simulink model "PKM_Planar_Testbench_2018"  (R2024a)
settings: Solver=FixedStepDiscrete  StartTime=0.0  StopTime=inf  FixedStep=param.t_sample  RelTol=1e-3
undefined symbols (not defined in the file or in its folder): max_qa, min_qa, param, slave3
libraries: Cust_Library_planarPKM x54, simulink_extras x27, dspswit3 x24, simulink x22, etherlab_lib x12
(part 3 of 6)

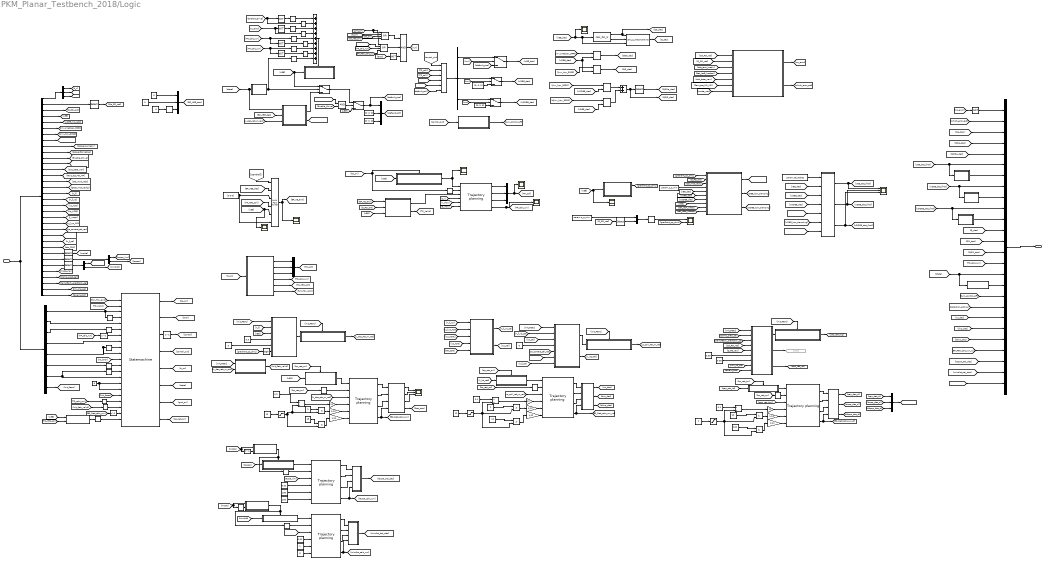
== system PKM_Planar_Testbench_2018/Logic ==
  note: Processing of logical signals
  note: xE: Desired platform pose
  note: Trajectory planning for activated inequality constraints
  note: Inverse kinematics
  note: Safety functions
  note: Platform Coordinate selection
  note: Structure opening for clamping contacts
  note: Retraction via contact coordinates
  note: Trajectory
  note: Check whether the EE target pose is in the operational space
      | and the corresponding joint angles are in the joint space
  note: Selection of the target EE pose for trajectoy planning
  note: For the PTP/CTP movement: An acceleration trapezoidal profile is calculated using the EE end target pose and the EE actual pose,
      | to determine the target EE pose, target EE velocity and target EE acceleration (all three in BP_target)
  note: Clamping reaction by platform reorientation
  note: Retraction movement via platform coordinates
  Data : Inport
  AND : Logic  AllPortsSameDT=off  OutDataTypeStr=boolean
  AND1 : Logic  Operator=OR  Inputs=4  AllPortsSameDT=off  OutDataTypeStr=boolean
  AND2 : Logic  Inputs=3  AllPortsSameDT=off  OutDataTypeStr=boolean
  AND3 : Logic  Operator=OR  Inputs=4  AllPortsSameDT=off  OutDataTypeStr=boolean
  Add : Sum  Inputs=9
  Add3 : Sum
  Angle clamping : Constant  Value=param.q_p_min  SampleTime=-1
  Angle clamping1 : Constant  Value=param.q_p_min  SampleTime=-1
  Bus Creator : BusCreator  Inputs=26
  Bus Selector : BusSelector  OutputSignals=Controlpanel.tv_vmax_amax,Kinematics_currentValues.Qa_rad_m,Kinematics_currentValues.Q_rad,Kinematics_currentValues.xEE_m_rad,Differential kinematics - current values.xDEE_ms_rads,Differential kinematics - current values.Jinv_hredqax,Differential kinematics - current values.Jinv_hqx,Differential kinematics - current values.dJinv_hqx,Differential kinematics - current values.det_JacA_hredx,Differential kinematics - current values.det_JacB_hredqa,Controlpanel.Enable_Drive,Controlpanel.Enable_PDControl,Beobachter.obs_beta_nan,Beobachter.rx,Differential kinematics - current values.QD_mod_rads,Differential kinematics - current values.QDD_mod_radss,Beobachter.Wirklinie_Fext_mP,Beobachter.Wirklinie_Fext_xp,Beobachter.xp_KS0,Beobachter.xp_KSGj,Beobachter.J_xpqa,Beobachter.n_f_xp_KS0,Beobachter.qa_contact_sel_rad,Beobachter.predbody_sel,Beobachter.n_f_qa,Controlpanel.retr_CS0,PD_Controller.mode_h_rrlevel_rrrueck,PD_Controller.kappa_lim_soll_ist,PD_Controller.min_dist_lim_soll_ist,PD_Controller.mode_nan,Beobachter.clamping_predicted,Beobachter.clampingChain_predicted,Differential kinematics - current values.Jinv_hqx_dq_dqa,Beobachter.tauext_obs
  Bus Selector1 : BusSelector  OutputSignals=Controlpanel.Drive_to_Position,Controlpanel.EMERGENCY_OFF,Controlpanel.GUI_started,State Variables.Controlword,Controlpanel.Drive_to_Homepose,Controlpanel.Enable_Drive,Controlpanel.Drive_trajectory,Beobachter.Init_Reaktion
  Clamping reaction : MATLAB Function  TreatAsAtomicUnit=on
  Constant : Constant  Value=[0;0;0]  SampleTime=-1
  Constant1 : Constant  Value=param.sel_redres  SampleTime=-1
  Constant10 : Constant  Value=150  SampleTime=-1
  Constant12 : Constant  Value=0  SampleTime=-1
  Constant14 : Constant  Value=150  SampleTime=-1
  Constant16 : Constant  SampleTime=-1
  Constant17 : Constant  Value=5  SampleTime=-1
  Constant18 : Constant  Value=0.01  SampleTime=-1
  Constant{4..5,7..8} (4 alike) : Constant  Value=[0; 0; 0]  SampleTime=-1
  Constant9 : Constant  Value=0.01  SampleTime=-1
  Degrees to Radians1 : simulink_extras/Transformations/Degrees to Radians
  Delay{,1..3,7,9,14..15} (8 alike) : Delay  DelayLength=1
  Demux1 : Demux  Outputs=2
  Demux2 : Demux  Outputs=2
  Demux3 : Demux  Outputs=3
  Demux4 : Demux  Outputs=3
  Divide : Product  Inputs=*/
  Divide1 : Product  Inputs=*/
  Divide2 : Product  Inputs=*/
  Edge Detector{1..6,8..21} (20 alike) : dspswit3/Edge Detector  InputProcessing=Columns as channels (frame based)
  Gain10 : Gain  Gain=12
  Gain{11..12,14..15,21..22} (6 alike) : Gain  Gain=1/12
  Gain13 : Gain  Gain=12
  Gain20 : Gain  Gain=12
  Goto106 : Goto  Commented=on  GotoTag=Jqap
  Gradient calculation : MATLAB Function  TreatAsAtomicUnit=on
  Hold Configuration after enabling1 : Subsystem  TreatAsAtomicUnit=on
  Hold Configuration after enabling2 : Subsystem  TreatAsAtomicUnit=on
  Hold Configuration after enabling3 : Subsystem  TreatAsAtomicUnit=on
  Hold Configuration after enabling4 : Subsystem  TreatAsAtomicUnit=on
  Hold Configuration after enabling5 : Subsystem  TreatAsAtomicUnit=on
  Hold Configuration after enabling6 : Subsystem  TreatAsAtomicUnit=on
  Hold Configuration after enabling7 : Subsystem  TreatAsAtomicUnit=on
  Hold Configuration after enabling8 : Subsystem  TreatAsAtomicUnit=on
  Hold Configuration after enabling9 : Subsystem  TreatAsAtomicUnit=on
  "Hold initial position as target value for PD_Controller " : Subsystem  TreatAsAtomicUnit=on
  MATLAB Function : MATLAB Function  TreatAsAtomicUnit=on
  MATLAB Function1 : MATLAB Function  TreatAsAtomicUnit=on
  MATLAB Function11 : MATLAB Function  TreatAsAtomicUnit=on
  MATLAB Function12 : MATLAB Function  TreatAsAtomicUnit=on
  MATLAB Function13 : MATLAB Function  TreatAsAtomicUnit=on
  MATLAB Function14 : MATLAB Function  TreatAsAtomicUnit=on
  MATLAB Function15 : MATLAB Function  TreatAsAtomicUnit=on
  MATLAB Function16 : MATLAB Function  TreatAsAtomicUnit=on
  MATLAB Function17 : MATLAB Function  TreatAsAtomicUnit=on
  MATLAB Function18 : MATLAB Function  TreatAsAtomicUnit=on
  MATLAB Function19 : MATLAB Function  TreatAsAtomicUnit=on
  MATLAB Function2 : MATLAB Function  TreatAsAtomicUnit=on
  MATLAB Function20 : MATLAB Function  TreatAsAtomicUnit=on
  MATLAB Function21 : MATLAB Function  TreatAsAtomicUnit=on
  MATLAB Function22 : MATLAB Function  TreatAsAtomicUnit=on
  MATLAB Function23 : MATLAB Function  TreatAsAtomicUnit=on
  MATLAB Function3 : MATLAB Function  TreatAsAtomicUnit=on
  MATLAB Function4 : MATLAB Function  TreatAsAtomicUnit=on
  MATLAB Function7 : MATLAB Function  TreatAsAtomicUnit=on
  MATLAB Function8 : MATLAB Function  TreatAsAtomicUnit=on
  MatrixMultiply{8..11} (4 alike) : Product  Multiplication=Matrix(*)
  Multiport Switch : MultiPortSwitch  Inputs=4  DataPortForDefault=Additional data port  DiagnosticForDefault=None  SaturateOnIntegerOverflow=off  InputSameDT=off
  Multiport Switch1 : MultiPortSwitch  Inputs=4  DataPortForDefault=Additional data port  DiagnosticForDefault=None  SaturateOnIntegerOverflow=off  InputSameDT=off
  Mux{,1,3..4,9} (5 alike) : Mux  Inputs=3
  Mux2 : Mux  Inputs=2
  NOT{,1..5} (6 alike) : Logic  Operator=NOT  AllPortsSameDT=off  OutDataTypeStr=boolean
  PHIE : Constant  Value=0  SampleTime=-1
  Radians to Degrees : simulink_extras/Transformations/Radians to Degrees
  Safety functions : Subsystem
  Saturation : Saturate  UpperLimit=12  LowerLimit=1
  Saturation1 : Saturate  UpperLimit=12  LowerLimit=1
  Saturation2 : Saturate  UpperLimit=12  LowerLimit=1
  Scope{,1,4,12,14,23,31} (7 alike) : Scope
  Scope27 : Scope  NumInputPorts=2
  Scope28 : Scope  NumInputPorts=3
  Scope48 : Scope  NumInputPorts=3
  Selector : Selector  InputPortWidth=9  IndexOptions=Index vector (dialog)  Indices=[2 5 8]  OutputSizes=1
  Selector2 : Selector  InputPortWidth=9  IndexOptions=Index vector (dialog)  Indices=[1 4 7]  OutputSizes=1
  Selector3 : Selector  InputPortWidth=4  IndexOptions=Index vector (dialog)  Indices=[1 2 3]  OutputSizes=1
  Selector5 : Selector  InputPortWidth=5  IndexOptions=Index vector (dialog)  Indices=[1]  OutputSizes=1
  Selector6 : Selector  InputPortWidth=4  IndexOptions=Index vector (dialog)  Indices=[1 4]  OutputSizes=1
  Selector7 : Selector  InputPortWidth=4  IndexOptions=Index vector (dialog)  Indices=[1 4]  OutputSizes=1
  Sign1 : Signum
  Statemachine : Cust_Library_planarPKM/Statemachine  SystemSampleTime=-1  VariantActivationTime=update diagram  AllowFlexibleInterface=on  Latency=0  AutoFrameSizeCalculation=off
  Switch{2..6} (5 alike) : Switch  Criteria=u2 > Threshold  SaturateOnIntegerOverflow=off  InputSameDT=off
  Trajectory : Subsystem
  Trajectory planning{,1..5} (6 alike) : Cust_Library_planarPKM/Trajectory planning
  Validation of the EE end target pose : Subsystem
  XE : Constant  Value=0  SampleTime=-1
  YE : Constant  Value=0  SampleTime=-1
  amax : Constant  Value=15  SampleTime=-1
  amax1 : Constant  Value=10  SampleTime=-1
  amax2 : Constant  Value=100  SampleTime=-1
  bp_rueck : Constant  Value=12  SampleTime=-1
  bp_rueck2 : Constant  Value=12  SampleTime=-1
  calc_full_ik : Cust_Library_planarPKM/calc_full_ik  psi_j=param.psi_j  beta_j=param.beta_j  r_fixPlat_j=param.r_fixPlat_j  r_mobPlat_j=param.r_mobPlat_j  l_all_id=param.l_all_id
  calc_q_rotConstraints : Cust_Library_planarPKM/calc_q_rotConstraints  psi_j=param.psi_j
  d_retr_cl1 : Constant  Value=0.05  SampleTime=-1
  d_retr_cl2 : Constant  Value=0.05  SampleTime=-1
  d_retr_m : Constant  Value=0.3  SampleTime=-1
  d_retr_m1 : Constant  Value=0  SampleTime=-1
  isStandstill : MATLAB Function  TreatAsAtomicUnit=on
  mult{,1..5} (6 alike) : Product  Inputs=**
  phi_retr_deg : Constant  Value=0  SampleTime=-1
  tp_retr1 : Constant  SampleTime=-1
  tv : Constant  Value=0.2  SampleTime=-1
  tv1 : Constant  Value=0.1  SampleTime=-1
  tv2 : Constant  Value=0.1  SampleTime=-1
  vmax : Constant  Value=2  SampleTime=-1
  vmax1 : Constant  Value=2  SampleTime=-1
  vmax2 : Constant  Value=20  SampleTime=-1
  Out1 : Outport
  wires:
  Data/1 -> Bus Selector/1, Bus Selector1/1
  [TP_Valid] -> Statemachine/2
  Bus Selector1/1 -> Statemachine/3, Edge Detector5/1  "<Drive_to_Position>"
  Bus Selector1/2 -> Statemachine/5  "<EMERGENCY_OFF>"
  [TP_calc_run] -> Delay/1
  Bus Selector1/4 -> Statemachine/8  "<Controlword>"
  Bus Selector1/5 -> Statemachine/10, Edge Detector6/1  "<Drive_to_Homepose>"
  Bus Creator/1 -> Out1/1  "Logical data"
  Delay/1 -> Statemachine/7  "bp_calc_run"
  [no_error] -> Statemachine/11  "err"
  [Qa_des] -> Bus Creator/3  "Qa_des_rad"
  [QDa_des] -> Bus Creator/4  "QDa_des_rads"
  [QDDa_des] -> Bus Creator/5  "QDDa_des_radss"
  [xEE_des_final] -> MATLAB Function/1(u), Bus Creator/6  "xEE_des_m_rad"
  [xDEE_des_final] -> MATLAB Function2/1(u), Bus Creator/8  "xDEE_des_ms_rads"
  [xDDEE_des_final] -> MATLAB Function3/1(u), Bus Creator/10  "xDDEE_des_mss_radss"
  [TP_calc_run] -> Bus Creator/15  "TP_isCalculating"
  [Q_des] -> Bus Creator/12  "Q_des_rad"
  [QD_des] -> Bus Creator/13  "QD_des_rads"
  [QDD_des] -> Bus Creator/14  "QDD_des_radss"
  Statemachine/1 -> [bp_on]  "bp_on"
  Statemachine/2 -> [error]  "error"
  Bus Selector/1 -> Demux3/1  "<tv_vmax_amax>"
  Demux3/1 -> [t_v]  "t_v"
  Demux3/2 -> [v_max]  "v_max"
  Demux3/3 -> [a_max]  "a_max"
  Bus Selector1/7 -> Statemachine/14, Edge Detector1/1  "<Drive_trajectory>"
  [TR_calc_run] -> Delay1/1
  Statemachine/5 -> [tr_on]  "tr_on"
  Delay1/1 -> Statemachine/18
  [xEE] -> MATLAB Function1/1(EE_act)
  [TR_XE0_soll] -> MATLAB Function1/2(vec_traj_0)
  [full_TR_valid] -> Statemachine/1
  Statemachine/4 -> [control_out]  "control_out"
  Statemachine/3 -> Delay3/1
  MATLAB Function1/1(TR_in_starting_pos) -> Delay2/1
  Delay2/1 -> Statemachine/21  "tr_in_starting_pos"
  Delay3/1 -> [control]  "control"
  Statemachine/6 -> [state]  "state"
  [state] -> isStandstill/1(u), Bus Creator/16  "state"
  Bus Selector/2 -> Selector3/1  "<Qa_rad_m>"
  Bus Selector1/3 -> Edge Detector4/1  "<GUI_started>"
  Edge Detector4/1 -> Statemachine/6  "GUI_started"
  Edge Detector5/1 -> Statemachine/4  "target_run_trig"
  Edge Detector6/1 -> Statemachine/9  "home_run_trig"
  Edge Detector1/1 -> Statemachine/13
  Bus Selector1/6 -> Edge Detector3/1  "<Enable_Drive>"
  Edge Detector3/1 -> Statemachine/12  "enable_drive"
  Mux4/1 -> [BP_XEE_des]
  PHIE/1 -> Degrees to Radians1/1
  Degrees to Radians1/1 -> Mux4/3
  YE/1 -> Mux4/2
  XE/1 -> Mux4/1
  Bus Selector/4 -> [xEE]  "<xEE_m_rad>"
  [control] -> Multiport Switch/1
  [BP_XEE_des] -> Multiport Switch/2
  Multiport Switch/1 -> [BP_XE_end], Scope12/1
  [TR_XE0_soll] -> Multiport Switch/4
  [xEE] -> Scope14/1, Multiport Switch/5
  Mux/1 -> Scope/1, [TP_soll]  "soll_BP"
  Validation of the EE end target pose/2(BP_valid) -> [TP_Valid]
  Trajectory planning/1 -> Mux/1
  [a_max] -> Trajectory planning/6
  Edge Detector2/1 -> Trajectory planning/2  "enable_bp"
  Hold Configuration after enabling1/1("vec_x_0_Startposition ") -> Trajectory planning/1, Scope4/1
  [t_v] -> Trajectory planning/4
  [bp_on] -> Hold Configuration after enabling1/Trigger, Edge Detector2/1  "enable_bp"
  [v_max] -> Trajectory planning/5
  [xEE] -> Hold Configuration after enabling1/1(Theta_ist)
  Validation of the EE end target pose/1(XE_end) -> Trajectory planning/3
  Trajectory planning/4 -> Scope23/1, [TP_calc_run]  "BP_isCalculating"
  [BP_XE_end] -> Validation of the EE end target pose/1(XE_soll_relab)
  Demux4/1 -> Switch3/1
  [default_pos] -> Switch3/3
  [run] -> Switch4/2
  [TP_soll] -> Multiport Switch1/2
  [TR_soll] -> Multiport Switch1/3
  Demux4/2 -> Switch4/1
  [default_soll] -> Multiport Switch1/6
  Demux4/3 -> Switch5/1
  [control_out] -> Multiport Switch1/1
  [run] -> Switch5/2
  [run] -> Switch3/2
  Multiport Switch1/1 -> Demux4/1
  Switch4/1 -> [xDEE_des]  "BP_XDE_soll"
  Switch3/1 -> [xEE_des]  "BP_XE_soll"
  Constant7/1 -> Switch4/3
  Switch5/1 -> [xDDEE_des]  "BP_XDDE_soll"
  Constant8/1 -> Switch5/3
  Trajectory/3(acc_soll) -> Mux1/3
  Trajectory/6(tr_valid) -> [full_TR_valid]
  Trajectory/1(pos_soll) -> Mux1/1
  Trajectory/4(tr_isCalculating) -> [TR_calc_run]
  Trajectory/5(XE0_soll) -> [TR_XE0_soll]
  [tr_on] -> Trajectory/1(tr_run)
  Mux1/1 -> [TR_soll]
  Trajectory/2(vel_soll) -> Mux1/2
  AND2/1 -> [run]
  [bp_on] -> AND3/3
  AND1/1 -> AND2/2
  [TR_calc_run] -> AND1/3
  NOT/1 -> AND2/3
  [error] -> NOT/1
  [tr_on] -> AND3/2
  [TP_calc_run] -> AND1/2
  AND3/1 -> AND2/1
  [xEE_des] -> Scope1/1, calc_q_rotConstraints/3, calc_full_ik/1
  calc_full_ik/2 -> calc_q_rotConstraints/2
  calc_q_rotConstraints/1 -> [Q_des]
  Add3/1 -> [QDD_des], Selector2/1
  [Jinv_hqx_3RRR] -> MatrixMultiply10/1
  [xDDEE_des] -> MatrixMultiply9/2
  MatrixMultiply11/1 -> Add3/2
  [xDEE_des] -> MatrixMultiply10/2, MatrixMultiply8/2
  [Jinv_hredqax_3RRR] -> MatrixMultiply8/1
  [xDEE_des] -> MatrixMultiply11/2
  MatrixMultiply9/1 -> Add3/1
  Selector3/1 -> [Qa_RD_rad]
  Safety functions/1(no_error) -> [no_error]  "err"
  [Qa_RD_rad] -> Safety functions/1(Qa_rad)
  Bus Selector/3 -> [Q_RD_rad]  "<Q_rad>"
  [Q_RD_rad] -> Safety functions/2(Q_ist_rad)
  MATLAB Function/1(y) -> Bus Creator/7  "xEE_des_m_rad_6D"
  MATLAB Function2/1(y) -> Bus Creator/9  "xDEE_des_ms_rads_6D"
  MATLAB Function3/1(y) -> Bus Creator/11  "xDDEE_des_mss_radss_6D"
  MatrixMultiply10/1 -> [QD_des]
  MatrixMultiply8/1 -> [QDa_des]
  Bus Selector/9 -> [det_JacA_hredx]  "<det_JacA_hredx>"
  Bus Selector/10 -> [det_JacB_hredqa]  "<det_JacB_hredqa>"
  [det_JacA_hredx] -> Safety functions/3(det_JacA_hredx_ist)
  [det_JacB_hredqa] -> Safety functions/4(det_JacB_hredqa_ist)
  [Enable_Drive] -> NOT2/1, Edge Detector9/1
  NOT1/1 -> Edge Detector15/1
  Edge Detector11/1 -> Add/4
  AND/1 -> Switch2/2
  Constant4/1 -> Mux3/2
  Edge Detector12/1 -> Add/5
  [Enable_Drive] -> AND/2
  Edge Detector15/1 -> Add/8
  [TP_calc_run] -> NOT1/1, Edge Detector10/1
  Switch6/1 -> Switch2/1
  Edge Detector14/1 -> Add/6
  Edge Detector10/1 -> Add/7
  Constant5/1 -> Mux3/3
  [no_error] -> Edge Detector11/1, NOT4/1
  Mux3/1 -> [default_soll]
  [TR_calc_run] -> NOT3/1, Edge Detector12/1
  Add/1 -> "Hold initial position as target value for PD_Controller "/Trigger
  [state] -> MATLAB Function13/1(state), MATLAB Function4/1(u)
  Edge Detector16/1 -> Add/9
  Edge Detector9/1 -> Add/2
  [Enable_PDControl] -> AND/1
  Edge Detector13/1 -> Add/3
  NOT4/1 -> Edge Detector13/1
  [xEE] -> Switch2/3
  [xEE] -> "Hold initial position as target value for PD_Controller "/1(Theta_ist), Switch6/1
  Switch2/1 -> [default_pos], Mux3/1
  NOT3/1 -> Edge Detector14/1
  MATLAB Function4/1(y) -> Edge Detector16/1, Switch6/2  "enable_bp"
  NOT2/1 -> Edge Detector8/1
  Edge Detector8/1 -> Add/1
  Bus Selector/11 -> [Enable_Drive]  "<Enable_Drive>"
  Bus Selector/12 -> [Enable_PDControl]  "<Enable_PDControl>"
  [no_error] -> NOT5/1
  NOT5/1 -> Bus Creator/1  "BP_isError"
  isStandstill/1(y) -> Bus Creator/17  "isStandstill"
  [Jinv_hqx_3RRR] -> MatrixMultiply9/1
  [dJinv_hqx_3RRR] -> MatrixMultiply11/1
  Selector2/1 -> [QDDa_des]
  Bus Selector/7 -> [Jinv_hqx_3RRR]  "<Jinv_hqx>"
  Bus Selector/8 -> [dJinv_hqx_3RRR]  "<dJinv_hqx>"
  Safety functions/2(which_error_act) -> [which_error_act]
  [which_error_act] -> Bus Creator/2  "which_error_act"
  Bus Selector/6 -> [Jinv_hredqax_3RRR]  "<Jinv_hredqax>"
  calc_full_ik/1 -> [Qa_des], calc_q_rotConstraints/1
  [control_out] -> MATLAB Function7/1(control_out)
  MATLAB Function7/1(turn_control_off) -> [turn_control_off]
  [turn_control_off] -> Bus Creator/18  "turn_control_off"
  Bus Selector/13 -> [obs_beta_nan]  "<obs_beta_nan>"
  [obs_beta_nan] -> Safety functions/5(obs_beta_nan)
  Bus Selector/14 -> [Fext_est_MO_MP]  "<rx>"
  [Fext_est_MO_MP] -> Safety functions/6(Fext_est_MO_MP)
  Selector/1 -> Mux2/2
  Mux2/1 -> Radians to Degrees/1
  [xEE_des] -> Clamping reaction/5(xEE_soll)
  [Q_RD_rad] -> Clamping reaction/2(q)
  [QD_mod_rads] -> Clamping reaction/3(dq)
  [xDEE_des] -> Clamping reaction/6(xDEE_soll)
  [xEE] -> Gradient calculation/1(xEE), Scope31/1
  [xDDEE_des] -> Clamping reaction/7(xDDEE_soll)
  Clamping reaction/1(xEE_korr) -> [xEE_korr_clamping]
  Gradient calculation/1(grad) -> [gradient_qp_phiz]
  Angle clamping/1 -> Clamping reaction/4(q_p_min)
  [xEE_des] -> MATLAB Function8/2(x_raw)
  [xDEE_des] -> MATLAB Function8/3(dx_raw)
  [xDDEE_des] -> MATLAB Function8/4(ddx_raw)
  [xDEE_korr_clamping] -> MATLAB Function8/6(dx_clamping)
  [xDDEE_korr_clamping] -> MATLAB Function8/7(ddx_clamping)
  [xEE_korr_clamping] -> MATLAB Function8/5(x_clamping)
  Constant1/1 -> MATLAB Function8/1(sel_redres)
  MATLAB Function8/1(x) -> Scope28/1, [xEE_des_final]
  MATLAB Function8/2(dx) -> Scope28/2, [xDEE_des_final]
  MATLAB Function8/3(ddx) -> Scope28/3, [xDDEE_des_final]
  Bus Selector/16 -> [QDD_mod_radss]  "<QDD_mod_radss>"
  Bus Selector/15 -> [QD_mod_rads]  "<QD_mod_rads>"
  Radians to Degrees/1 -> Scope27/1
  [Q_RD_rad] -> Validation of the EE end target pose/2(Q_ist_rad)
  [xEE] -> Validation of the EE end target pose/3(xEE_ist_m_rad)
  Constant12/1 -> Statemachine/16, Statemachine/15
  [GMT_soll] -> Multiport Switch1/4
  Statemachine/7 -> [gmt_on]
  [gmt_on] -> AND3/1, AND1/1
  Bus Selector/5 -> [xDEE_ms_rads]  "<xDEE_ms_rads>"
  Bus Selector1/8 -> [Init_Reac]  "<Init_Reaktion>"
  Bus Selector/17 -> [n_f]  "<Wirklinie_Fext_mP>"
  Constant/1 -> Multiport Switch/6, Multiport Switch/3
  Hold Configuration after enabling2/1("x_ist_retr_trigg ") -> [x_des_retr_m_rad]
  [n_f] -> MATLAB Function11/2(n_f)
  [Init_Reac] -> MATLAB Function11/1(Init_Reaction)
  [xEE] -> MATLAB Function11/3(x)
  MATLAB Function11/1(x_des_retr_m_rad) -> Hold Configuration after enabling2/1(x_ist_retr)
  [Init_Reac] -> Hold Configuration after enabling2/Trigger
  [x_des_retr_m_rad] -> MATLAB Function12/2(x_soll_retr_m_rad)
  [Init_Reac] -> MATLAB Function12/1(Init_Reac)
  MATLAB Function12/1(Init_Retr_valid) -> [Init_Retr_valid]
  [Init_Retr_valid] -> Delay7/1
  Delay7/1 -> Statemachine/19
  Hold Configuration after enabling3/1("vec_x_0_Startposition ") -> Trajectory planning1/1
  Trajectory planning1/1 -> MATLAB Function21/1(s_in_)
  Trajectory planning1/4 -> [BP_Retr_calc_run], MATLAB Function21/4(trigger)
  Gain14/1 -> Trajectory planning1/5
  Gain15/1 -> Trajectory planning1/6
  Edge Detector17/1 -> Trajectory planning1/2  "enable_bp"
  [x_des_retr_m_rad] -> Trajectory planning1/3
  [bp_retr_on] -> Edge Detector17/1  "enable_bp"
  [BP_Retr_calc_run] -> Delay9/1
  [BP_Retr_calc_run] -> AND1/4
  [Retr_des] -> Multiport Switch1/5
  Delay9/1 -> Statemachine/20
  tv/1 -> Divide1/1
  Statemachine/8 -> [bp_retr_on]
  [bp_retr_on] -> AND3/4
  Trajectory planning1/2 -> MATLAB Function21/2(v_in_)
  Trajectory planning1/3 -> MATLAB Function21/3(a_in_)
  [xEE] -> Hold Configuration after enabling3/1(Theta_ist)
  [BP_XEE_des] -> MATLAB Function13/2(x_des_bp)
  [x_des_retr_m_rad] -> MATLAB Function13/3(x_des_retr)
  MATLAB Function13/1(y) -> Switch6/3
  MATLAB Function13/2(retraction_active) -> [retraction_active]
  [retraction_active] -> Bus Creator/19  "retraction_active"
  Trajectory planning/2 -> Mux/2
  Trajectory planning/3 -> Mux/3
  d_retr_m/1 -> MATLAB Function11/4(d_retr_m)
  Clamping reaction/3(xDDEE_korr) -> [xDDEE_korr_clamping]
  Clamping reaction/2(xDEE_korr) -> [xDEE_korr_clamping]
  [det_JacA_hredx] -> Clamping reaction/9(det_JacA)
  [det_JacB_hredqa] -> Clamping reaction/10(det_JacB)
  [gradient_qp_phiz] -> Sign1/1
  Sign1/1 -> MATLAB Function11/6(sign_grad_qp_phiz)
  phi_retr_deg/1 -> MATLAB Function11/5(phi_retr_deg)
  Bus Selector/18 -> [n_f_xp]  "<Wirklinie_Fext_xp>"
  Bus Selector/19 -> [xp_KS0]  "<xp_KS0>"
  d_retr_m1/1 -> MATLAB Function14/4(d_rueckz_m)
  [Init_Reac] -> Hold Configuration after enabling4/Trigger
  MATLAB Function14/1(x_soll_retr_m_rad) -> Hold Configuration after enabling4/1(x_ist_retr)
  [xp_sel] -> MATLAB Function14/3(x_ist)
  [Init_Reac] -> MATLAB Function14/1(Init_Reaktion)
  [n_f_xp_sel] -> MATLAB Function14/2(n_f)
  Hold Configuration after enabling4/1("x_ist_retr_trigg ") -> [xp_soll_retr_m_rad]
  [x_ist_retr] -> Hold Configuration after enabling5/1(Theta_ist)
  Trajectory planning2/3 -> MATLAB Function15/3(a_in)
  Trajectory planning2/2 -> MATLAB Function15/2(v_in)
  tv1/1 -> Divide/1
  [bp_retr_on] -> Hold Configuration after enabling5/Trigger  "enable_bp"
  [xp_soll_retr_m_rad] -> Trajectory planning2/3
  Edge Detector18/1 -> Trajectory planning2/2
  amax1/1 -> mult1/1
  vmax1/1 -> mult/1
  Trajectory planning2/4 -> [BP_Retr_calc_run_xp], MATLAB Function15/4(trigger)
  Trajectory planning2/1 -> MATLAB Function15/1(s_in)
  Hold Configuration after enabling5/1("vec_x_0_Startposition ") -> Trajectory planning2/1
  [xp_des] -> Bus Creator/20  "xp_des"
  [dxp_des] -> Bus Creator/21  "dxp_des"
  [ddxp_des] -> Bus Creator/22  "ddxp_des"
  Bus Selector/20 -> [xp_KSGj]  "<xp_KSGj>"
  Bus Selector/21 -> [J_xpqa]  "<J_xpqa>"
  [BP_Retr_calc_run_xp] -> Bus Creator/23  "BP_Retr_calc_run_xp"
  MATLAB Function15/1(s_out) -> [xp_des]
  MATLAB Function15/2(v_out) -> [dxp_des]
  MATLAB Function15/3(a_out) -> [ddxp_des]
  Bus Selector/22 -> [n_f_xp_KS0]  "<n_f_xp_KS0>"
  [n_f_xp_KS0] -> MATLAB Function16/2(n_f_xp_KS0)
  [xp_KS0] -> MATLAB Function16/4(xp_KS0)
  MATLAB Function16/2(xp_sel) -> [xp_sel]
  MATLAB Function16/1(n_f_xp_sel) -> [n_f_xp_sel]
  [xp_KSGj] -> MATLAB Function16/3(xp_KSGj)
  [n_f_xp] -> MATLAB Function16/1(n_f_xp)
  Bus Selector/23 -> [qa_contact_sel_rad]  "<qa_contact_sel_rad>"
  Bus Selector/24 -> [predbody_sel]  "<predbody_sel>"
  [qa_contact_sel_rad] -> MATLAB Function14/5(qa_contact_sel_rad)
  [predbody_sel] -> MATLAB Function14/6(predbody)
  Bus Selector/25 -> [n_f_qa]  "<n_f_qa>"
  [n_f_qa] -> MATLAB Function14/7(n_f_qa)
  MATLAB Function14/2(x_ist_retr) -> [x_ist_retr]
  Bus Selector/26 -> [retr_CS0]  "<retr_CS0>"
  [retr_CS0] -> MATLAB Function16/5(rueck_KS0)
  Gain10/1 -> Trajectory planning2/4
  Divide/1 -> Gain10/1
  bp_rueck2/1 -> Saturation/1
  Gain11/1 -> Trajectory planning2/5
  Gain12/1 -> Trajectory planning2/6
  mult/1 -> Gain11/1
  mult1/1 -> Gain12/1
  Saturation/1 -> Divide/2, mult/2, mult1/2
  Saturation1/1 -> mult3/2, Divide1/2, mult2/2
  mult3/1 -> Gain15/1
  mult2/1 -> Gain14/1
  Divide1/1 -> Gain13/1
  Gain13/1 -> Trajectory planning1/4
  vmax/1 -> mult2/1
  amax/1 -> mult3/1
  bp_rueck/1 -> Saturation1/1
  Bus Selector/27 -> Selector5/1  "<mode_h_rrlevel_rrrueck>"
  Selector5/1 -> [mode]
  Bus Selector/28 -> Selector6/1  "<kappa_lim_soll_ist>"
  Bus Selector/29 -> Selector7/1  "<min_dist_lim_soll_ist>"
  Selector6/1 -> Demux1/1
  Selector7/1 -> Demux2/1
  Demux1/1 -> [kappa_lim]
  Demux1/2 -> [kappa]
  Demux2/2 -> [mindist]
  Demux2/1 -> [mindist_lim]
  Trajectory planning5/3 -> MATLAB Function19/3(a_in)
  Trajectory planning5/2 -> MATLAB Function19/2(v_in)
  Trajectory planning5/4 -> MATLAB Function19/4(trigger), [kappa_calc_run]
  Constant10/1 -> Trajectory planning5/5
  Constant9/1 -> Trajectory planning5/4
  Hold Configuration after enabling6/1("vec_x_0_Startposition ") -> Trajectory planning5/1
  Edge Detector19/1 -> Trajectory planning5/2  "enable_bp"
  Constant14/1 -> Trajectory planning5/6
  Trajectory planning5/1 -> MATLAB Function19/1(s_in)
  MATLAB Function19/1(out) -> [kappa_traj_des]
  MATLAB Function17/1(y) -> Hold Configuration after enabling6/Trigger, Edge Detector19/1
  [mode] -> Delay14/1, MATLAB Function17/1(mode)
  [kappa] -> Hold Configuration after enabling6/1(Theta_ist)
  [kappa_lim] -> Trajectory planning5/3
  Delay14/1 -> MATLAB Function17/2(mode_prev)
  Delay15/1 -> MATLAB Function18/2(mode_prev)
  [mindist_lim] -> Trajectory planning4/3
  [mindist] -> Hold Configuration after enabling7/1(Theta_ist)
  [mode] -> MATLAB Function18/1(mode), Delay15/1
  MATLAB Function18/1(y) -> Hold Configuration after enabling7/Trigger, Edge Detector20/1
  MATLAB Function20/1(out) -> [mindist_traj_des]
  Trajectory planning4/1 -> MATLAB Function20/1(s_in)
  Constant17/1 -> Trajectory planning4/6
  Edge Detector20/1 -> Trajectory planning4/2  "enable_bp"
  Hold Configuration after enabling7/1("vec_x_0_Startposition ") -> Trajectory planning4/1
  Constant18/1 -> Trajectory planning4/4
  Constant16/1 -> Trajectory planning4/5
  Trajectory planning4/4 -> [mindist_calc_run], MATLAB Function20/4(trigger)
  Trajectory planning4/2 -> MATLAB Function20/2(v_in)
  Trajectory planning4/3 -> MATLAB Function20/3(a_in)
  [kappa_traj_des] -> Bus Creator/24  "kappa_traj_des"
  [mindist_traj_des] -> Bus Creator/25  "mindist_traj_des"
  MATLAB Function21/1(s_out) -> Scope48/1
  MATLAB Function21/3(a_out) -> Scope48/3
  MATLAB Function21/4(retr_soll) -> [Retr_des]  "soll_BP"
  MATLAB Function21/2(v_out) -> Scope48/2
  Bus Selector/30 -> [mode_nan]  "<mode_nan>"
  [mode_nan] -> Safety functions/7(mode_nan)
  Bus Selector/31 -> [clamp_pred_sel]  "<clamping_predicted>"
  Bus Selector/32 -> [clampBody_predbody_sel]  "<clampingChain_predicted>"
  [clamp_pred_sel] -> MATLAB Function22/2(clamping_det)
  [clampBody_predbody_sel] -> MATLAB Function22/3(clampBody)
  [Qa_RD_rad] -> MATLAB Function22/4(qa)
  [Q_RD_rad] -> MATLAB Function22/5(q)
  [Init_Reac] -> MATLAB Function22/1(Init_reaction)
  d_retr_cl1/1 -> MATLAB Function22/6(d_retr_cl1)
  [Jinv_hq_qa] -> MATLAB Function22/8(Jinv_hq_qa)
  Bus Selector/33 -> [Jinv_hq_qa]  "<Jinv_hqx_dq_dqa>"
  MATLAB Function22/1(qap_retr_soll) -> Hold Configuration after enabling8/1(qap_retr)
  Hold Configuration after enabling8/1("qap_retr_trig ") -> [qap_retr_trig]
  MATLAB Function22/2(J_qap) -> Goto106/1
  Saturation2/1 -> mult5/2, mult4/2, Divide2/2
  mult5/1 -> Gain22/1
  mult4/1 -> Gain21/1
  Gain22/1 -> Trajectory planning3/6
  Gain21/1 -> Trajectory planning3/5
  tp_retr1/1 -> Saturation2/1
  Divide2/1 -> Gain20/1
  Gain20/1 -> Trajectory planning3/4
  MATLAB Function23/3(a_out) -> [ddqap_des_cl]
  MATLAB Function23/2(v_out) -> [dqap_des_cl]
  MATLAB Function23/1(s_out) -> [qap_des_cl]
  Hold Configuration after enabling9/1("vec_x_0_Startposition ") -> Trajectory planning3/1
  Trajectory planning3/1 -> MATLAB Function23/1(s_in)
  Trajectory planning3/4 -> MATLAB Function23/4(trigger), [BP_Retr_calc_run_cl]
  vmax2/1 -> mult4/1
  amax2/1 -> mult5/1
  Edge Detector21/1 -> Trajectory planning3/2
  [qap_retr_trig] -> Trajectory planning3/3
  [bp_retr_on] -> Hold Configuration after enabling9/Trigger
  tv2/1 -> Divide2/1
  Trajectory planning3/2 -> MATLAB Function23/2(v_in)
  Trajectory planning3/3 -> MATLAB Function23/3(a_in)
  [qap_retr_ist] -> Hold Configuration after enabling9/1(Theta_ist)
  MATLAB Function22/3(qap_retr) -> [qap_retr_ist]
  [dqap_des_cl] -> Mux9/2
  [ddqap_des_cl] -> Mux9/3
  [qap_des_cl] -> Mux9/1
  Mux9/1 -> [traj_qap_des_cl]
  [traj_qap_des_cl] -> Bus Creator/26  "traj_qap_soll_cl"
  Bus Selector/34 -> [tauext_obs]  "<tauext_obs>"
  [tauext_obs] -> MATLAB Function22/9(tauext_obs)
  [Init_Reac] -> Hold Configuration after enabling8/Trigger
  [gradient_qp_phiz] -> Scope27/2
  [gradient_qp_phiz] -> Clamping reaction/1(grad)
  [xEE] -> Clamping reaction/8(xEE_ist)
  Angle clamping1/1 -> Mux2/1
  [Q_RD_rad] -> Selector/1
  [bp_retr_on] -> Hold Configuration after enabling3/Trigger  "enable_bp"
  [bp_retr_on] -> Edge Detector18/1
  d_retr_cl2/1 -> MATLAB Function22/7(d_retr_cl2)
  [bp_retr_on] -> Edge Detector21/1
  [Init_Reac] -> Statemachine/17

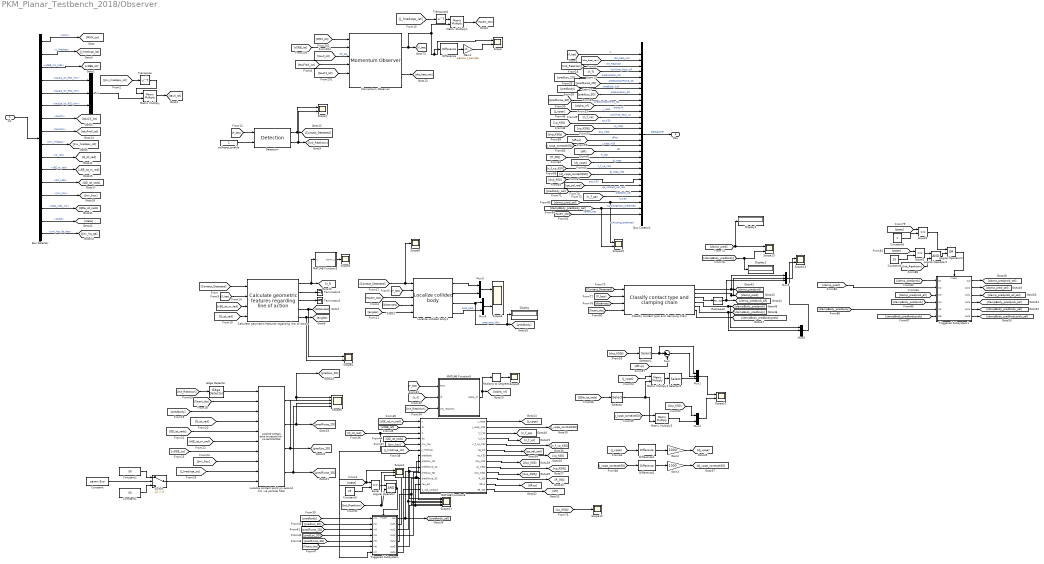
== system PKM_Planar_Testbench_2018/Observer ==
  In1 : Inport
  Bus Creator1 : BusCreator  Inputs=29
  Bus Selector : BusSelector  OutputSignals=Dynamik.MMX,Differential kinematics - current values.J_hredxqa,Differential kinematics - current values.xDEE_ms_rads,Messdaten.tauQa_ist_RD1_Nm,Messdaten.tauQa_ist_RD2_Nm,Messdaten.tauQa_ist_RD3_Nm,Dynamik.tauCX,Dynamik.tauFraX,Differential kinematics - current values.Jinv_hredqax,Kinematics_currentValues.Q_rad,Kinematics_currentValues.xEE_m_rad,Differential kinematics - current values.QD_rads,Differential kinematics - current values.Jinv_hqx,Differential kinematics - current values.QDa_rads_ms,Logical data.state,Differential kinematics - current values.Jinv_hqx_dq_dqa
  Calculate geometric features regarding line of action : Cust_Library_planarPKM/Calculate geometric features regarding line of action  psi_j=param.psi_j  r_fixPlat_j=param.r_fixPlat_j  l_all_id=param.l_all_id
  Classify contact type and clamping chain : Cust_Library_planarPKM/Classify contact type and clamping chain  ffnn_clamping_param=param.ffnn_clamping_param  ffnn_clamping_chain_param=param.ffnn_clamping_chain_param
  Constant : Constant  Value=param.Exp  SampleTime=-1
  Constant1 : Constant  Value=50  SampleTime=-1
  Constant2 : Constant  Value=50  SampleTime=-1
  Constant3 : Constant  Value=25  SampleTime=-1
  Constant4 : Constant  Value=25  SampleTime=-1
  Constant6 : Constant  SampleTime=-1
  Detection : Cust_Library_planarPKM/Detection  ColDet_thresholds=param.CollDet_limit_MobPlat_soft
  Difference : simulink/Discrete/Difference  ICPrevInput=zeros(3,1)  OutMin=[]  OutMax=[]  OutDataType=fixdt(1, 16)  OutScaling=2^-10  DoSatur=off
  Difference1 : simulink/Discrete/Difference  ICPrevInput=zeros(3,3)  OutMin=[]  OutMax=[]  OutDataType=fixdt(1, 16)  OutScaling=2^-10  DoSatur=off
  Difference2 : simulink/Discrete/Difference  ICPrevInput=zeros(3,3)  OutMin=[]  OutMax=[]  OutDataType=fixdt(1, 16)  OutScaling=2^-10  DoSatur=off
  Display : Display
  Display1 : Display
  Display2 : Display
  Edge Detector : dspswit3/Edge Detector  InputProcessing=Columns as channels (frame based)
  Equal : RelationalOperator  Operator===  OutDataTypeStr=boolean  RndMeth=Simplest  InputSameDT=off
  Equal1 : RelationalOperator  Operator===  OutDataTypeStr=boolean  RndMeth=Simplest  InputSameDT=off
  Equal2 : RelationalOperator  Operator===  OutDataTypeStr=boolean  RndMeth=Simplest  InputSameDT=off
  Gain1 : Gain  Gain=param.t_sample
  Gain2 : Gain  Gain=1000
  Gain3 : Gain  Gain=1000
  Localize collided body1 : Cust_Library_planarPKM/Localize collided body  min_dist_threshold=param.min_dist_threshold  min_angle_threshold_deg=param.min_angle_threshold_deg  min_torque_threshold=param.min_torque_threshold  ffnn_ClCollB_param=param.ffnn_ClCollB_param
  Localize contact point on second link via particle filter : Cust_Library_planarPKM/Localize contact point on second link via particle filter  pf_dim=param.pf_dim  l_all=param.l_all  r_BasisPla_MobPla=param.r_BasisPla_MobPla  l_all_id=param.l_all_id  r_fixPlat_j=param.r_fixPlat_j  r_mobPlat_j=param.r_mobPlat_j  psi_j=param.psi_j  x_N_2D=param.x_N_2D  x_CovR_Inv_2D=param.x_CovR_Inv_2D  x_N_3D=param.x_N_3D  x_CovR_Inv_3D=param.x_CovR_Inv_3D
  Logical Operator : Logic  AllPortsSameDT=off  OutDataTypeStr=boolean
  Logical Operator1 : Logic  AllPortsSameDT=off  OutDataTypeStr=boolean
  Logical Operator2 : Logic  Operator=OR  AllPortsSameDT=off  OutDataTypeStr=boolean
  MATLAB Function3 : MATLAB Function  TreatAsAtomicUnit=on
  MATLAB Function5 : MATLAB Function  TreatAsAtomicUnit=on
  MATLAB Function6 : MATLAB Function  TreatAsAtomicUnit=on
  Matrix Multiply{,1..3} (4 alike) : Product  Multiplication=Matrix(*)
  Momentum Observer : Cust_Library_planarPKM/Momentum Observer  Ko=param.Kox  t_sample=param.t_sample  initial_Fext=zeros(3,1)
  Mux{,1,5..6} (4 alike) : Mux  Inputs=3
  Mux2 : Mux  Inputs=2
  Mux3 : Mux  Inputs=2
  Mux4 : Mux  Inputs=2
  Radians to Degrees : simulink_extras/Transformations/Radians to Degrees
  Reshape3 : Reshape
  Scope{,3..4,7,10,13..15} (8 alike) : Scope  NumInputPorts=2
  Scope1 : Scope  NumInputPorts=3
  Scope11 : Scope  NumInputPorts=6
  Scope{5..6,9,12} (4 alike) : Scope
  Scope8 : Scope  NumInputPorts=4
  Selector : Selector  InputPortWidth=4  IndexOptions=Index vector (dialog)  Indices=[1 2 3]  OutputSizes=1
  Selector1 : Selector  InputPortWidth=3  IndexOptions=Index vector (dialog)  Indices=[1 2]  OutputSizes=1
  Selector2 : Selector  InputPortWidth=3  IndexOptions=Index vector (dialog)  Indices=[1 2]  OutputSizes=1
  Sum : Sum  Inputs=|+-
  Switch : Switch  Criteria=u2 > Threshold  SaturateOnIntegerOverflow=off  InputSameDT=off
  Terminator1 : Terminator
  Terminator2 : Terminator
  Transpose : Math  Operator=transpose  SignedPower=on
  Transpose1 : Math  Operator=transpose  SignedPower=on
  Triggered Subsystem : Subsystem  TreatAsAtomicUnit=on
  Triggered Subsystem1 : Subsystem  TreatAsAtomicUnit=on
  collreact_enable : Constant  SampleTime=-1
  Obs : Outport
  wires:
  Bus Selector/8 -> [tauFraX_ist]  "<tauFraX>"
  Bus Selector/9 -> [Jinv_hredqax_ist]  "<Jinv_hredqax>"
  Bus Selector/2 -> [J_hredxqa_ist]  "<J_hredxqa>"
  Bus Creator1/1 -> Obs/1  "Beobachter"
  Bus Selector/1 -> [MMX_ist]  "<MMX>"
  In1/1 -> Bus Selector/1
  Bus Selector/3 -> [xDEE_ist]  "<xDEE_ms_rads>"
  Bus Selector/4 -> Mux/1  "<tauQa_ist_RD1_Nm>"
  Bus Selector/5 -> Mux/2  "<tauQa_ist_RD2_Nm>"
  Bus Selector/6 -> Mux/3  "<tauQa_ist_RD3_Nm>"
  Mux/1 -> Matrix Multiply/2
  [Jinv_hredqax_ist] -> Transpose/1
  Transpose/1 -> Matrix Multiply/1
  Matrix Multiply/1 -> [tauX_ist]
  [F_beo] -> Bus Creator1/1  "rx"
  Bus Selector/7 -> [tauCX_ist]  "<tauCX>"
  Bus Selector/10 -> [Q_ist_rad]  "<Q_rad>"
  [obs_beta_nan] -> Bus Creator1/2  "obs_beta_nan"
  Bus Selector/11 -> [xEE_ist_m_rad]  "<xEE_m_rad>"
  [J_hredxqa_ist] -> Transpose1/1
  Transpose1/1 -> Matrix Multiply1/1
  [F_beo] -> Calculate geometric features regarding line of action/2
  [Q_ist_rad] -> Calculate geometric features regarding line of action/4
  [xEE_ist_m_rad] -> Calculate geometric features regarding line of action/3
  Matrix Multiply1/1 -> [Tauext_obs]
  [Tauext_obs] -> Localize collided body1/3
  [F_beo] -> Localize collided body1/2
  Calculate geometric features regarding line of action/1 -> MATLAB Function3/1(u), [n_f]
  Calculate geometric features regarding line of action/2 -> Terminator1/1
  Calculate geometric features regarding line of action/3 -> Terminator2/1
  Calculate geometric features regarding line of action/4 -> Scope4/1, [distances]
  Calculate geometric features regarding line of action/5 -> Scope4/2, [angles]
  [distances] -> Localize collided body1/4
  [angles] -> Localize collided body1/5
  collreact_enable/1 -> Detection/2
  [F_beo] -> Detection/1
  Detection/1 -> Scope7/1, [Contact_Detected]
  [Init_Reaktion] -> Bus Creator1/3  "Init_Reaktion"
  [n_f] -> Bus Creator1/4  "Wirklinie_Fext_mP"
  [Contact_Detected] -> Localize collided body1/1, Scope6/1
  MATLAB Function3/1(norm_u) -> Scope5/1
  Detection/2 -> Scope7/2, [Init_Reaktion]
  Bus Selector/12 -> [QD_ist_rads]  "<QD_rads>"
  [J_hredxqa_ist] -> Localize contact point on second link via particle filter/9
  [xDEE_ist] -> Localize contact point on second link via particle filter/7
  [QD_ist_rads] -> Localize contact point on second link via particle filter/5
  [Q_ist_rad] -> Localize contact point on second link via particle filter/4
  [predbody] -> Localize contact point on second link via particle filter/3
  [Tauext_obs] -> Localize contact point on second link via particle filter/2
  [xEE_ist_m_rad] -> Localize contact point on second link via particle filter/6
  Localize contact point on second link via particle filter/1 -> [predLoc_2D], Scope8/1
  Localize contact point on second link via particle filter/2 -> Scope8/3, [predForce_2D]
  [predLoc_2D] -> Bus Creator1/5  "predLocation_2D"
  [predForce_2D] -> Bus Creator1/6  "predContactForce_2D"
  Bus Selector/13 -> [Jinv_hqx]  "<Jinv_hqx>"
  [Jinv_hqx] -> Localize contact point on second link via particle filter/8
  [predbody] -> Bus Creator1/7  "predBody_Coll"
  Localize contact point on second link via particle filter/3 -> Scope8/2, [predLoc_3D]
  Localize contact point on second link via particle filter/4 -> Scope8/4, [predForce_3D]
  [predLoc_3D] -> Bus Creator1/8  "predLocation_3D"
  [predForce_3D] -> Bus Creator1/9  "predContactForce_3D"
  Difference/1 -> Gain1/1
  Gain1/1 -> Scope/2
  [F_beo] -> MATLAB Function5/1(Fext)
  [n_f] -> MATLAB Function5/2(nf)
  MATLAB Function5/1(alpha_nf) -> Radians to Degrees/1, [alpha_nf]
  [alpha_nf] -> Bus Creator1/10  "alpha_nf"
  Radians to Degrees/1 -> Scope9/1
  [Init_Reaktion] -> MATLAB Function5/3(init_reaction)
  [xEE_ist_m_rad] -> MATLAB Function6/1(x)
  [Q_ist_rad] -> Triggered Subsystem/7(In7), MATLAB Function6/3(q)
  [Jinv_hqx] -> MATLAB Function6/5(Jinv_hqx)
  [J_hredxqa_ist] -> MATLAB Function6/6(J_hredxqa)
  [xDEE_ist] -> MATLAB Function6/2(dx)
  [QD_ist_rads] -> MATLAB Function6/4(dq)
  MATLAB Function6/1(J_xpqa) -> [J_xpqa]
  MATLAB Function6/4(n_f_xp) -> [n_f_xp]
  [n_f_xp] -> Bus Creator1/12  "Wirklinie_Fext_xp"
  [J_xpqa] -> Bus Creator1/11  "J_xpqa"
  MATLAB Function6/7(xp_KS0) -> [xp_KS0]
  [xp_KS0] -> Bus Creator1/13  "xp_KS0"
  MATLAB Function6/9(xp_KSGj) -> [xp_KSGj]
  [xp_KSGj] -> Bus Creator1/14  "xp_KSGj"
  [predbody] -> Triggered Subsystem/1(In1)
  [predLoc_2D] -> Triggered Subsystem/2(In2)
  [predForce_2D] -> Triggered Subsystem/3(In3)
  [predLoc_3D] -> Triggered Subsystem/4(In4)
  [predForce_3D] -> Triggered Subsystem/5(In5)
  [Tauext_obs] -> Triggered Subsystem/6(In6)
  Triggered Subsystem/1(out) -> MATLAB Function6/7(predbody), Scope11/1, [predbody_sel]
  Triggered Subsystem/2(out1) -> MATLAB Function6/8(predLoc_2D), Scope11/2
  Triggered Subsystem/3(out2) -> MATLAB Function6/9(predForce_2D), Scope11/3
  Triggered Subsystem/4(out3) -> MATLAB Function6/10(predLoc_3D), Scope11/4
  Triggered Subsystem/5(out4) -> MATLAB Function6/11(predForce_3D), Scope11/5
  Triggered Subsystem/6(out5) -> MATLAB Function6/12(tau_ext), Scope11/6
  [Init_Reaktion] -> Scope1/2, Logical Operator/2
  MATLAB Function6/8(dxp_KS0) -> [dxp_KS0]
  MATLAB Function6/10(dxp_KSGj) -> [dxp_KSGj]
  MATLAB Function6/2(J_xpqa_KS0) -> [J_xpqa_contactKS0]
  Bus Selector/14 -> [QDa_ist_rads]  "<QDa_rads_ms>"
  [J_xpqa] -> Matrix Multiply2/1
  [J_xpqa_contactKS0] -> Matrix Multiply3/1
  [QDa_ist_rads] -> Selector/1
  Matrix Multiply2/1 -> Selector2/1
  [dxp_KS0] -> Mux2/1
  Matrix Multiply3/1 -> Mux2/2
  Mux1/1 -> Scope10/1
  Mux2/1 -> Scope10/2
  Selector/1 -> Matrix Multiply3/2, Matrix Multiply2/2
  MATLAB Function6/12(dRxp) -> [dRxp]
  [dxp_KSGj] -> Selector1/1
  [dRxp] -> Sum/2
  Sum/1 -> Mux1/2
  Selector1/1 -> Mux1/1, Sum/1
  Selector2/1 -> Mux1/3
  [dxp_KSGj] -> Bus Creator1/15  "dxp_KSGj"
  [dRxp] -> Bus Creator1/16  "dRxp"
  [J_xpqa_contactKS0] -> Bus Creator1/17  "J_xpqa_KS0"
  MATLAB Function6/13(dR_0Gj) -> [dR]
  [dR] -> Bus Creator1/18  "dR"
  MATLAB Function6/11(R_0Gj) -> [R_0Gj]
  [R_0Gj] -> Bus Creator1/19  "R_0Gj"
  [Init_Reaktion] -> Edge Detector/1
  Edge Detector/1 -> Localize contact point on second link via particle filter/1
  [J_xpqa] -> Difference1/1
  Difference1/1 -> Gain2/1
  Gain2/1 -> [dJ_xpqa]
  [dJ_xpqa] -> Bus Creator1/20  "dJ_xpqa"
  MATLAB Function6/5(n_f_xp_KS0) -> [n_f_xp_KS0]
  [n_f_xp_KS0] -> Bus Creator1/21  "n_f_xp_KS0"
  Gain3/1 -> [dJ_xpqa_contactKS0]
  Difference2/1 -> Gain3/1
  [J_xpqa_contactKS0] -> Difference2/1
  [dJ_xpqa_contactKS0] -> Bus Creator1/22  "dJ_xpqa_KS0"
  [dxp_KS0] -> Bus Creator1/23  "dxp_KS0"
  Triggered Subsystem/7(out6) -> MATLAB Function6/13(q_rad_contact)
  MATLAB Function6/6(qa_sel) -> [qa_sel_rad]
  [qa_sel_rad] -> Bus Creator1/24  "qa_contact_sel_rad"
  [predbody_sel] -> Bus Creator1/25  "predbody_sel"
  MATLAB Function6/3(n_f_qa) -> [n_f_qa]
  [n_f_qa] -> Bus Creator1/26  "n_f_qa"
  [xp_KSGj] -> Scope12/1
  Localize collided body1/1 -> Mux3/1
  Localize collided body1/2 -> Mux3/2
  Mux3/1 -> Scope3/1
  Localize collided body1/3 -> Mux4/1, Display/1, [predbody]  "pred_body_ffnn"
  Localize collided body1/4 -> Mux4/2  "pred_body"
  Mux4/1 -> Scope3/2
  [Contact_Detected] -> Calculate geometric features regarding line of action/1
  Switch/1 -> Localize contact point on second link via particle filter/10
  Constant/1 -> Switch/2
  Constant1/1 -> Switch/3
  Constant2/1 -> Switch/1
  Bus Selector/15 -> [state]  "<state>"
  [state] -> Scope1/1, Equal/1
  Equal/1 -> Logical Operator/1
  Constant3/1 -> Equal/2
  Logical Operator/1 -> Scope1/3, Triggered Subsystem/Trigger
  [Contact_Detected] -> Classify contact type and clamping chain/1
  [distances] -> Classify contact type and clamping chain/3
  [F_beo] -> Classify contact type and clamping chain/2
  Classify contact type and clamping chain/1 -> Mux5/1, [clamp_predprob]
  Classify contact type and clamping chain/2 -> Mux5/2, [clamp_pred]
  Classify contact type and clamping chain/4 -> Mux6/1, [clampBody_predprob]
  Classify contact type and clamping chain/5 -> Mux6/2, [clampBody_predbody]
  Reshape3/1 -> [clamp_predprob_all], Mux5/3
  Mux5/1 -> Scope14/1
  Mux6/1 -> Scope14/2
  [clamp_pred] -> Display1/1, Scope13/1
  [clampBody_predbody] -> Display2/1, Scope13/2
  Logical Operator2/1 -> Triggered Subsystem1/Trigger
  Constant4/1 -> Equal1/2
  Equal1/1 -> Logical Operator1/1
  [state] -> Equal1/1
  [Init_Reaktion] -> Logical Operator1/2
  [clamp_predprob] -> Triggered Subsystem1/1(In1)
  [clamp_pred] -> Triggered Subsystem1/2(In2)
  [clamp_predprob_all] -> Triggered Subsystem1/3(In3)
  [clampBody_predprob] -> Triggered Subsystem1/4(In4)
  [clampBody_predbody] -> Triggered Subsystem1/5(In5)
  [clampBody_predbodyprob] -> Triggered Subsystem1/6(In6)
  Triggered Subsystem1/6(out5) -> [clampBody_predbodyprob_sel]
  Triggered Subsystem1/5(out4) -> [clampBody_predbody_sel]
  Triggered Subsystem1/4(out3) -> [clampBody_predprob_sel]
  Triggered Subsystem1/3(out2) -> [clamp_predprob_all_sel]
  Triggered Subsystem1/2(out1) -> [clamp_pred_sel]
  Triggered Subsystem1/1(out) -> [clamp_predprob_sel]
  [clamp_pred_sel] -> Scope15/1, Bus Creator1/27  "clamping_predicted"
  [clampBody_predbody_sel] -> Scope15/2, Bus Creator1/28  "clampingChain_predicted"
  Bus Selector/16 -> [Jinv_hq_qa]  "<Jinv_hqx_dq_dqa>"
  [Tauext_obs] -> Bus Creator1/29  "tauext_obs"
  Logical Operator1/1 -> Logical Operator2/2
  [state] -> Equal2/1
  Constant6/1 -> Equal2/2
  Equal2/1 -> Logical Operator2/1
  [Tauext_obs] -> Classify contact type and clamping chain/4
  Momentum Observer/1 -> Scope/1, Difference/1, Matrix Multiply1/2, [F_beo]
  [MMX_ist] -> Momentum Observer/1
  [xDEE_ist] -> Momentum Observer/2
  [tauX_ist] -> Momentum Observer/3  "de_Qa"
  [tauFraX_ist] -> Momentum Observer/4
  [tauCX_ist] -> Momentum Observer/5
  Momentum Observer/2 -> [obs_beta_nan]
  Classify contact type and clamping chain/3 -> Reshape3/1
  Classify contact type and clamping chain/6 -> [clampBody_predbodyprob]
  ? -> Momentum Observer/6
